simulink model "complete_plant"  (R2022a)
settings: Solver=VariableStepAuto  StartTime=0.0  StopTime=15  RelTol=1e-3
values from neighbouring files (symbols this model uses):
  a = Simulink.Parameter(1.14)    [startup.m]
  A1 = Simulink.Parameter(39.8344)    [startup.m]
  A2 = Simulink.Parameter(813.0780)    [startup.m]
  b = Simulink.Parameter(-0.03291)    [startup.m]
  B1 = Simulink.Parameter(0.000001287)    [startup.m]
  B2 = Simulink.Parameter(-0.002325)    [startup.m]
  B3 = Simulink.Parameter(3.797)    [startup.m]
  c = Simulink.Parameter(-1.14)    [startup.m]
  C1 = Simulink.Parameter(-0.000000002541)    [startup.m]
  C2 = Simulink.Parameter(0.000005279)    [startup.m]
  C3 = Simulink.Parameter(-0.003943)    [startup.m]
  C4 = Simulink.Parameter(3.634)    [startup.m]
  C_param = Simulink.Parameter([0 13757.41 21278.97 26666.02 30253.47 30313.18 30313.18])    [startup.m]
  d = Simulink.Parameter(-1.027)    [startup.m]
  driver_gain = 0.4    [startup.m]
  FZ_C = Simulink.Parameter([0 204.13 427.04 668.1 895.72 1124.40 1324.40])    [startup.m]
  gr = Simulink.Parameter([6.63043, 6.63043, 7.95652, 7.95652])    [startup.m]
  I = 15    [startup.m]
  inch2mm = Simulink.Parameter(25.4)    [startup.m]
  J_z = Simulink.Parameter(75)    [startup.m]
  k_limit = Simulink.Parameter(3.461)    [startup.m]
  Ku = Simulink.Parameter(0.24 / g.Value)    [startup.m]
  l = Simulink.Parameter([0.7922471, 0.7828529])    [startup.m]
  max_yaw_field = Simulink.Parameter([1.34 1.34 1.34 1.66 1.14 1.24 0.754 0.849 0.85 0.85])    [startup.m]
  min_speed_regen = Simulink.Parameter(85)    [startup.m]
  motor_efficiency = Simulink.Parameter([0.85, 0.85, 0.85, 0.85])    [startup.m]
  motor_limit_power = Simulink.Parameter([0, 0, 15000, 15000])    [startup.m]
  motor_limit_torque = Simulink.Parameter([-25, 25])    [startup.m]
  mu_factor = Simulink.Parameter(2/3)    [startup.m]
  P = 1    [startup.m]
  RE = Simulink.Parameter(0.2228169203)    [startup.m]
  s = Simulink.Parameter([0.647895, 0.62102])    [startup.m]
  S1 = Simulink.Parameter(7 * (10^(-5)))    [startup.m]
  S2 = Simulink.Parameter(-0.0038)    [startup.m]
  S3 = Simulink.Parameter(0.6535)    [startup.m]
  S4 = Simulink.Parameter(0.1061)    [startup.m]
  steer_slope = Simulink.Parameter(0.0111)    [startup.m]
  T = 0    [startup.m]
  T2F = Simulink.Parameter(single([29 29 35 35]))    [startup.m]
  tau = Simulink.Parameter(0)    [startup.m]
  time_delay = 0.022    [startup.m]
  V_target = Simulink.Parameter([0 3 6 9 12 15 18 21 25 31])    [startup.m]
undefined symbols (not defined in the file or in its folder): Ag, brake_pressure, DiscIntNeverNeededParam, driver_input, FZ, omega, power_limits, psi, rdot, shock_displacement, shock_velocity, steering_angle, Vg, y, yaw
libraries: fl_lib x20, nesl_utility x12, sdl_lib x4, slpidlib x2, autolibdatasheetbattery x1, autolibmappedmotor x1, vehdynlibtire x1, simulink x1, autolibshared x1, vehdynlibviscommon x1
(part 2 of 3)

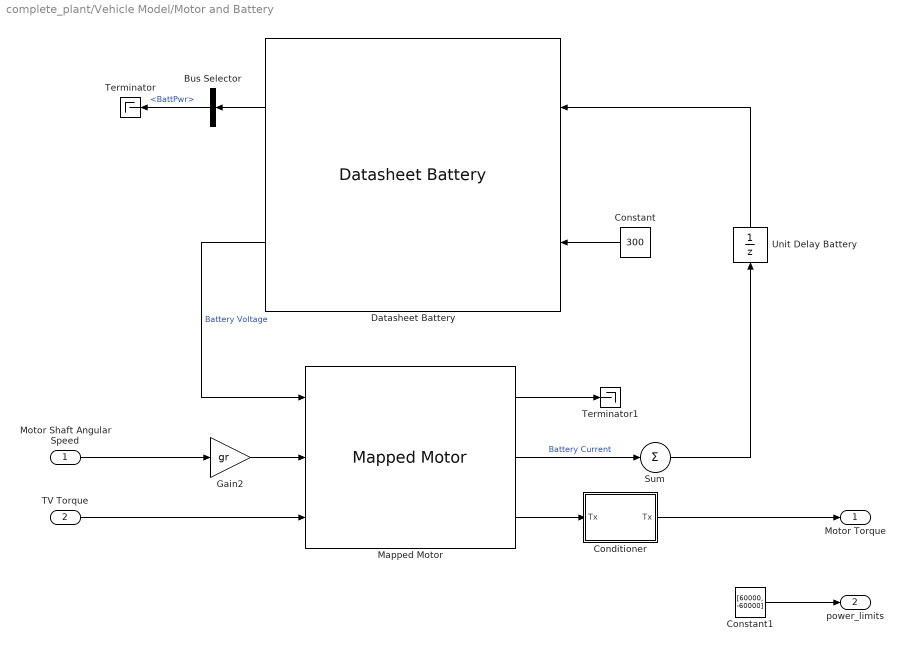
== system complete_plant/Vehicle Model/Motor and Battery ==
  Motor Shaft Angular Speed : Inport
  TV Torque : Inport  Port=2
  Bus Selector : BusSelector  OutputSignals=BattPwr
  Conditioner : MATLAB Function  TreatAsAtomicUnit=on  SystemSampleTime=0.0005
  Constant : Constant  Value=300
  Constant1 : Constant  Value=[60000, -60000]
  Datasheet Battery : autolibdatasheetbattery/Datasheet Battery  CapacityCtrl=Parameter  OutputVlt=Unfiltered  BattChargeMax=16  Em=[2.8 3.228 3.284 3.361 3.408 3.427 3.472 3.477 3.493 3.504 3.516 3.528 3.537 3.545 3.555 3.561 3.566 3.576 3.587 3.589 3.594 3.6 3.608 3.61 3.616 3.619 3.626 3.632 3.637 3.64 3.645 3.646 3.652 3.655 3.658 3.661 3.664 3.668 3.673 3.678 3.68 3.681 3.686 3.692 3.699 3.702 3.705 3.71 3.717 3.723 3.728 3.733 3.735 3.742 3.749 3.755 3.761 3.768 3.773 3.78 3.791 3.798 3.798 3.814 3.818 3.825 3.841 3.846 3.855 3.863 3.877 3.885 3.894 3.907 3.919 3.926 3.935 3.944 3.954 3.964 3.974 3.988 3.998 4.014 4.029 4.034 4.047 4.065 4.074 4.086 4.097 4.131 4.126 4.138 4.15 4.18 4.174 4.187 4.207 4.231 4.221]  CapLUTBp=[0 0.01 0.02 0.03 0.04 0.05 0.06 0.07 0.08 0.09 0.1 0.11 0.12 0.13 0.14 0.15 0.16 0.17 0.18 0.19 0.2 0.21 0.22 0.23 0.24 0.25 0.26 0.27 0.28 0.29 0.3 0.31 0.32 0.33 0.34 0.35 0.36 0.37 0.38 0.39 0.4 0.41 0.42 0.43 0.44 0.45 0.46 0.47 0.48 0.49 0.5 0.51 0.52 0.53 0.54 0.55 0.56 0.57 0.58 0.59 0.6 0.61 0.62 0.63 0.64 0.65 0.66 0.67 0.68 0.69 0.7 0.71 0.72 0.73 0.74 0.75 0.76 0.77 0.78 0.79 0.8 0.81 0.82 0.83 0.84 0.85 0.86 0.87 0.88 0.89 0.9 0.91 0.92 0.93 0.94 0.95 0.96 0.97 0.98 0.99 1]  RInt=[0.008846 0.009319 0.009027 0.00847 0.01032 0.01314;0.006389 0.006554 0.005553 0.005525 0.006043 0.007805;0.004364 0.004101 0.00406 0.003452 0.003846 0.004517;0.002031 0.002563 0.002532 0.00246 0.002716 0.003047;0.001443 0.001825 0.001795 0.001778 0.001924 0.002234;0.0005603 0.0007192 0.0006887 0.0007557 0.0007355 0.001014;0.001028 0.001338 0.001 0.001536 0.001546 0.002789]  BattTempBp=[243.1 253.1 263.1 273.1 283.1 298.1 313.1]  CapSOCBp=[0 0.2 0.4 0.6 0.8 1]  Ns=80  Np=4  BattCapInit=16  Tc=1/1000  Vinit=4.221  RefBlkName='autolibdatasheetbattery/Datasheet Battery'
      settings: SourceProductBaseCode=PW
  Gain2 : Gain  Gain=gr
  Mapped Motor : autolibmappedmotor/Mapped Motor  port_config=Speed  param_by=Tabulated torque-speed envelope  w_t=max_rpm  T_t=max_torque  torque_max=.1  power_max=30  Tc=0.002  param_loss=Tabulated efficiency data  eff=100  w_eff=375  T_eff=0.08  Piron=0  Pbase=0  w_eff_bp=rpm_sweep  T_eff_bp=torque_sweep  Temp_eff_bp=[233.15 293.15 373.15]  losses_table=[1.49 1.67 2.21 3.10; 0.42 0.69 1.14 2.03; 0.06 0.24 0.78 1.68; 0.42 0.69 1.14 2.03; 1.49 1.67 2.21 3.10]  losses_table_3d=cat(3,[1.49 1.67 2.21 3.10; 0.42 0.69 1.14 2.03; 0.06 0.24 0.78 1.68; 0.42 0.69 1.14 2.03; 1.49 1.67 2.21 3.10],[1.49 1.67 2.21 3.10; 0.42 0.69 1.14 2.03; 0.06 0.24 0.78 1.68; 0.42 0.69 1.14 2.03; 1.49 1.67 2.21 3.10],[1.49 1.67 2.21 3.10; 0.42 0.69 1.14 2.03; 0.06 0.24 0.78 1.68; 0.42 0.69 1.14 2.03; 1.49 1.67 2.21 3.10])  efficiency_table=efficiency_grid  efficiency_table_3d=cat(3,[95 95 95 95; 95 95 95 95; 95 95 95 95; 95 95 95 95; 95 95 95 95],[95 95 95 95; 95 95 95 95; 95 95 95 95; 95 95 95 95; 95 95 95 95],[95 95 95 95; 95 95 95 95; 95 95 95 95; 95 95 95 95; 95 95 95 95])  J=5e-6  b=1e-5  omega_o=0  T_t_extended=[0 0.947 1.252 1.562 1.875 2.191 2.511 2.834 3.161 3.491 3.824 4.16 4.499 4.84 5.185 5.532 5.882 6.234 6.589 6.946 7.305 7.666 8.029 8.395 8.762 9.131 9.501 10.247 10.622 10.999 11.376 11.755 12.135 12.516 12.897 13.28 13.663 14.047 14.431 14.815 15.2 15.586 15.971 16.356 16.742 17.127 17.512 17.897 18.281 18.665 19.048 19.431 19.813 20.194 20.574 20.953 21.331 21.708 22.084 22.458 22.83 23.202 23.571 23.939 24.305 24.669 25 25 25 24.669 24.305 23.939 23.571 23.202 22.83 22.458 22.084 21.708 21.331 20.953 20.574 20.194 19.813 19.431 19.048 18.665 18.281 17.897 17.512 17.127 16.742 16.356 15.971 15.586 15.2 14.815 14.431 14.047 13.663 13.28 12.897 12.516 12.135 11.755 11.376 10.999 10.622 10.247 9.501 9.131 8.762 8.395 8.029 7.666 7.305 6.946 6.589 6.234 5.882 5.532 5.185 4.84 4.499 4.16 3.824 3.491 3.161 2.834 2.511 2.191 1.875 1.562 1.252 0.947 0]  w_t_extended=[-1138.429400556 -1112.773060581 -1105.8091968735 -1098.950052921 -1092.2165726745 -1085.5982841585 -1079.095187373 -1072.6968103425 -1066.4136250425 -1060.2351594975 -1054.1614137075 -1048.202859648 -1042.3490253435 -1036.5894388185 -1030.945044024 -1025.394897009 -1019.9389977735 -1014.587818293 -1009.330886592 -1004.1682026705 -999.0997665285 -994.125578166 -989.245637583 -984.449472804 -979.7475558045 -975.129414609 -970.5950492175 -961.7776458465 -957.494607867 -953.2953456915 -949.1693873445 -945.116732826 -941.1478541115 -937.2522792255 -933.4195361925 -929.6705689635 -925.9844335875 -922.37160204 -918.832074321 -915.355378455 -911.941514442 -908.590482282 -905.302281975 -902.076913521 -898.9039049445 -895.793728221 -892.735911375 -889.740926382 -886.7983012665 -883.9080360285 -881.070130668 -878.2741132095 -875.5304556285 -872.839157925 -870.1897481235 -867.582226224 -865.0165922265 -862.492846131 -860.0109879375 -857.571017646 -855.162463281 -852.795796818 -850.4605462815 -848.1567116715 -845.8947649635 -843.6537622065 -841.626809470934 0 841.626809470934 843.6537622065 845.8947649635 848.1567116715 850.4605462815 852.795796818 855.162463281 857.571017646 860.0109879375 862.492846131 865.0165922265 867.582226224 870.1897481235 872.839157925 875.5304556285 878.2741132095 881.070130668 883.9080360285 886.7983012665 889.740926382 892.735911375 895.793728221 898.9039049445 902.076913521 905.302281975 908.590482282 911.941514442 915.355378455 918.832074321 922.37160204 925.9844335875 929.6705689635 933.4195361925 937.2522792255 941.1478541115 945.116732826 949.1693873445 953.2953456915 957.494607867 961.7776458465 970.5950492175 975.129414609 979.7475558045 984.449472804 989.245637583 994.125578166 999.0997665285 1004.1682026705 1009.330886592 1014.587818293 1019.9389977735 1025.394897009 1030.945044024 1036.5894388185 1042.3490253435 1048.202859648 1054.1614137075 1060.2351594975 1066.4136250425 1072.6968103425 1079.095187373 1085.5982841585 1092.2165726745 1098.950052921 1105.8091968735 1112.773060581 1138.429400556]  KLossIron=0  KLossCopper=0  x_w_eff_vec=[-1110.029403 -1099.5574275 -1089.085452 -1078.6134765 -1068.141501 -1057.6695255 -1047.19755 -1036.7255745 -1026.253599 -1015.7816235 -1005.309648 -994.8376725 -984.365697 -973.8937215 -963.421746 -952.9497705 -942.477795 -932.0058195 -921.533844 -911.0618685 -900.589893 -890.1179175 -879.645942 -869.1739665 -858.701991 -848.2300155 -837.75804 -827.2860645 -816.814089 -806.3421135 -795.870138 -785.3981625 -774.926187 -764.4542115 -753.982236 -743.5102605 -733.038285 -722.5663095 -712.094334 -701.6223585 -691.150383 -680.6784075 -670.206432 -659.7344565 -649.262481 -638.7905055 -628.31853 -617.8465545 -607.374579 -596.9026035 -586.430628 -575.9586525 -565.486677 -555.0147015 -544.542726 -534.0707505 -523.598775 -513.1267995 -502.654824 -492.1828485 -481.710873 -471.2388975 -460.766922 -450.2949465 -439.822971 -429.3509955 -418.87902 -408.4070445 -397.935069 -387.4630935 -376.991118 -366.5191425 -356.047167 -345.5751915 -335.103216 -324.6312405 -314.159265 -303.6872895 -293.215314 -282.7433385 -272.271363 -261.7993875 -251.327412 -240.8554365 -230.383461 -219.9114855 -209.43951 -198.9675345 -188.495559 -178.0235835 -167.551608 -157.0796325 -146.607657 -136.1356815 -125.663706 -115.1917305 -104.719755 -94.2477795 -83.775804 -73.3038285 -62.831853 -52.3598775 -41.887902 -31.4159265 -20.943951 -10.4719755 0 10.4719755 20.943951 31.4159265 41.887902 52.3598775 62.831853 73.3038285 83.775804 94.2477795 104.719755 115.1917305 125.663706 136.1356815 146.607657 157.0796325 167.551608 178.0235835 188.495559 198.9675345 209.43951 219.9114855 230.383461 240.8554365 251.327412 261.7993875 272.271363 282.7433385 293.215314 303.6872895 314.159265 324.6312405 335.103216 345.5751915 356.047167 366.5191425 376.991118 387.4630935 397.935069 408.4070445 418.87902 429.3509955 439.822971 450.2949465 460.766922 471.2388975 481.710873 492.1828485 502.654824 513.1267995 523.598775 534.0707505 544.542726 555.0147015 565.486677 575.9586525 586.430628 596.9026035 607.374579 617.8465545 628.31853 638.7905055 649.262481 659.7344565 670.206432 680.6784075 691.150383 701.6223585 712.094334 722.5663095 733.038285 743.5102605 753.982236 764.4542115 774.926187 785.3981625 795.870138 806.3421135 816.814089 827.2860645 837.75804 848.2300155 858.701991 869.1739665 879.645942 890.1179175 900.589893 911.0618685 921.533844 932.0058195 942.477795 952.9497705 963.421746 973.8937215 984.365697 994.8376725 1005.309648 1015.7816235 1026.253599 1036.7255745 1047.19755 1057.6695255 1068.141501 1078.6134765 1089.085452 1099.5574275 1110.029403]  x_T_eff_vec=[-25 -24.9 -24.8 -24.7 -24.6 -24.5 -24.4 -24.3 -24.2 -24.1 -24 -23.9 -23.8 -23.7 -23.6 -23.5 -23.4 -23.3 -23.2 -23.1 -23 -22.9 -22.8 -22.7 -22.6 -22.5 -22.4 -22.3 -22.2 -22.1 -22 -21.9 -21.8 -21.7 -21.6 -21.5 -21.4 -21.3 -21.2 -21.1 -21 -20.9 -20.8 -20.7 -20.6 -20.5 -20.4 -20.3 -20.2 -20.1 -20 -19.9 -19.8 -19.7 -19.6 -19.5 -19.4 -19.3 -19.2 -19.1 -19 -18.9 -18.8 -18.7 -18.6 -18.5 -18.4 -18.3 -18.2 -18.1 -18 -17.9 -17.8 -17.7 -17.6 -17.5 -17.4 -17.3 -17.2 -17.1 -17 -16.9 -16.8 -16.7 -16.6 -16.5 -16.4 -16.3 -16.2 -16.1 -16 -15.9 -15.8 -15.7 -15.6 -15.5 -15.4 -15.3 -15.2 -15.1 -15 -14.9 -14.8 -14.7 -14.6 -14.5 -14.4 -14.3 -14.2 -14.1 -14 -13.9 -13.8 -13.7 -13.6 -13.5 -13.4 -13.3 -13.2 -13.1 -13 -12.9 -12.8 -12.7 -12.6 -12.5 -12.4 -12.3 -12.2 -12.1 -12 -11.9 -11.8 -11.7 -11.6 -11.5 -11.4 -11.3 -11.2 -11.1 -11 -10.9 -10.8 -10.7 -10.6 -10.5 -10.4 -10.3 -10.2 -10.1 -10 -9.9 -9.8 -9.7 -9.6 -9.5 -9.4 -9.3 -9.2 -9.1 -9 -8.9 -8.8 -8.7 -8.6 -8.5 -8.4 -8.3 -8.2 -8.1 -8 -7.9 -7.8 -7.7 -7.6 -7.5 -7.4 -7.3 -7.2 -7.1 -7 -6.9 -6.8 -6.7 -6.6 -6.5 -6.4 -6.3 -6.2 -6.1 -6 -5.9 -5.8 -5.7 -5.6 -5.5 -5.4 -5.3 -5.2 -5.1 -5 -4.9 -4.8 -4.7 -4.6 -4.5 -4.4 -4.3 -4.2 -4.1 -4 -3.9 -3.8 -3.7 -3.6 -3.5 -3.4 -3.3 -3.2 -3.1 -3 -2.9 -2.8 -2.7 -2.6 -2.5 -2.4 -2.3 -2.2 -2.1 -2 -1.9 -1.8 -1.7 -1.6 -1.5 -1.4 -1.3 -1.2 -1.1 -1 -0.9 -0.8 -0.7 -0.6 -0.5 -0.4 -0.3 -0.2 -0.1 0 0.1 0.2 0.3 0.4 0.5 0.6 0.7 0.8 0.9 1 1.1 1.2 1.3 1.4 1.5 1.6 1.7 1.8 1.9 2 2.1 2.2 2.3 2.4 2.5 2.6 2.7 2.8 2.9 3 3.1 3.2 3.3 3.4 3.5 3.6 3.7 3.8 3.9 4 4.1 4.2 4.3 4.4 4.5 4.6 4.7 4.8 4.9 5 5.1 5.2 5.3 5.4 5.5 5.6 5.7 5.8 5.9 6 6.1 6.2 6.3 6.4 6.5 6.6 6.7 6.8 6.9 7 7.1 7.2 7.3 7.4 7.5 7.6 7.7 7.8 7.9 8 8.1 8.2 8.3 8.4 8.5 8.6 8.7 8.8 8.9 9 9.1 9.2 9.3 9.4 9.5 9.6 9.7 9.8 9.9 10 10.1 10.2 10.3 10.4 10.5 10.6 10.7 10.8 10.9 11 11.1 11.2 11.3 11.4 11.5 11.6 11.7 11.8 11.9 12 12.1 12.2 12.3 12.4 12.5 12.6 12.7 12.8 12.9 13 13.1 13.2 13.3 13.4 13.5 13.6 13.7 13.8 13.9 14 14.1 14.2 14.3 14.4 14.5 14.6 14.7 14.8 14.9 15 15.1 15.2 15.3 15.4 15.5 15.6 15.7 15.8 15.9 16 16.1 16.2 16.3 16.4 16.5 16.6 16.7 16.8 16.9 17 17.1 17.2 17.3 17.4 17.5 17.6 17.7 17.8 17.9 18 18.1 18.2 18.3 18.4 18.5 18.6 18.7 18.8 18.9 19 19.1 19.2 19.3 19.4 19.5 19.6 19.7 19.8 19.9 20 20.1 20.2 20.3 20.4 20.5 20.6 20.7 20.8 20.9 21 21.1 21.2 21.3 21.4 21.5 21.6 21.7 21.8 21.9 22 22.1 22.2 22.3 22.4 22.5 22.6 22.7 22.8 22.9 23 23.1 23.2 23.3 23.4 23.5 23.6 23.7 23.8 23.9 24 24.1 24.2 24.3 24.4 24.5 24.6 24.7 24.8 24.9 25]  x_tmp_eff_vec=[-0.09 -0.06 -0.03 0 0.03 0.06 0.09]  x_losses_mat=[2840.43469490031 2805.54744132541 2779.87827049912 2755.63794377818 2733.28147280803 2711.85439946791 2691.24197140587 2671.58877513259 2653.09092346246 2635.0273221516 2618.00782766042 2602.75353700982 2587.04654178768 2572.24579661788 2557.8249286228 2543.77817688114 2530.89179302846 2518.30507115493 2506.11534821342 2494.39397053384 2483.42163017641 2473.65854517521 2463.97979007223 2454.19251617385 2444.74900186613 2434.38941762584 2424.02577848989 2418.02563977851 2412.06569218952 2404.29517518479 2397.44512723314 2390.85220674868 2384.60553603402 2378.95108104658 2373.53020217171 2368.28006687239 2363.00734989155 2358.1662204294 2353.3050369761 2349.21895724092 2345.2633086809 2341.72012007622 2338.58679501067 2335.3809658645 2333.42741875647 2331.43827917154 2329.38942604396 2327.36890336757 2325.26286477187 2323.15588643422 2321.85279256551 2320.45569086905 2318.96446325893 2318.07546934648 2317.46979216667 2316.76053101971 2315.94754163419 2315.93163246198 2316.05712329708 2316.06870267075 2315.96619495001 2316.10738282262 2316.66145037877 2317.09334863559 2317.40287478073 2317.58982555269 2318.21339083604 2319.53316070594 2320.71785979788 2321.76723845613 2322.68104640929 2323.45903276846 2325.03910278562 2327.01714211556 2328.84573681222 2330.52457939056 2332.05336152146 2333.43177402878 2334.6595068864 2336.99421292983 2339.33774137948 2341.51697955451 2343.53155456892 2345.38109240743 2347.06521792118 2348.58355482343 2349.93572568528 2352.56915552233 2355.22622344414 2357.70089624007 2359.99271294185 2362.10121102651 2364.02592640988 2365.76639344001 2367.3221448905 2368.69271195385 2370.28402549494 2373.03179176203 2375.57628226626 2377.91692391904 2380.05314147556 2381.98435752456 2383.70999247813 2385.22946456146 2386.54218980253 2387.64758202168 2388.54505282122 2389.2340115749 2390.39858396493 2392.57021654128 2394.51210477741 2396.22352041458 2397.70373211284 2398.95200543468 2399.96760282866 2400.7497836128 2401.29780395804 2401.61091687151 2401.6883721796 2401.52941651112 2401.13329328017 2400.49924266899 2399.62650161072 2399.31691235657 2400.01959760851 2400.45785502685 2400.63073258304 2400.5372736729 2400.17651708907 2399.5474969933 2398.64924288848 2397.48077959063 2396.04112720045 2394.32930107483 2392.34431179814 2390.08516515324 2387.55086209234 2384.74039870762 2381.6527662016 2378.28695085743 2374.64193400878 2370.71669200961 2366.51019620374 2364.01151523306 2361.45747055781 2358.58844286227 2355.40311978209 2351.90018165219 2348.07830145599 2343.9361447741 2339.47236973265 2334.68562695117 2329.57455948998 2324.13780279725 2318.37398465549 2312.28172512768 2305.85963650287 2299.10632324142 2292.02038191968 2284.60040117421 2276.8449616456 2268.75263592173 2260.32198848061 2251.55157563268 2242.43994546265 2232.98563777082 2223.1871840139 2213.04310724539 2202.55192205531 2192.53352715951 2183.39290654335 2173.8616545439 2163.93786292719 2153.61961101 2142.90496555821 2131.7919806841 2120.2786977426 2108.36314522666 2096.04333866144 2083.31728049752 2070.18296000306 2056.63835315487 2042.68142252842 2028.3101171867 2013.52237256806 1998.31611037286 1982.689238449 1966.63965067636 1950.16522684997 1933.26383256213 1915.93331908323 1898.1715232415 1879.97626730137 1861.34535884079 1842.27659062714 1822.76774049201 1802.81657120464 1782.42083034405 1761.57825016994 1740.28654749222 1718.54342353919 1696.34656382443 1673.69363801224 1650.5822997818 1627.01018668981 1602.9749200318 1578.47410470199 1553.91013607881 1530.09128917938 1505.73387899734 1480.83467203205 1455.39040884597 1429.39780380407 1402.85354481015 1375.75429303985 1348.09668267054 1319.87732060787 1291.09278620896 1261.73963100229 1231.81437840412 1201.3135234314 1170.23353241123 1138.57084268672 1106.32186231915 1073.4829697866 1040.05051367869 1006.02081238763 971.390153795415 936.154794957117 900.310961780193 863.854848699832 826.782618350201 789.090401231568 750.774295373247 711.830365992272 672.254645147765 632.043131390936 ...(+1787558 chars)]  x_losses_mat_3d=[37.8947368421052 25.2631578947368 12.6315789473684 0 12 24 36;18.9473684210526 12.6315789473684 6.3157894736842 0 5.99999999999999 12 18;0 0 0 0 0 0 0;18 12 5.99999999999999 0 6.3157894736842 12.6315789473684 18.9473684210526;36 24 12 0 12.6315789473684 25.2631578947368 37.8947368421052]  CalLossMapData={}  CalLossWithTempMapData={}  aMode=1  RefBlkName='autolibmappedmotor/Mapped Motor'
      settings: SourceProductBaseCode=PW,DR,MT,VE
  Sum : Sum  Inputs=+
  Terminator : Terminator
  Terminator1 : Terminator
  Unit Delay Battery : UnitDelay  SampleTime=0.0005  HasFrameUpgradeWarning=on
  Motor Torque : Outport
  power_limits : Outport  Port=2
  wires:
  Datasheet Battery/1 -> Bus Selector/1
  Constant/1 -> Datasheet Battery/2
  Unit Delay Battery/1 -> Datasheet Battery/1
  Datasheet Battery/2 -> Mapped Motor/1  "Battery Voltage"
  TV Torque/1 -> Mapped Motor/3
  Motor Shaft Angular Speed/1 -> Gain2/1
  Gain2/1 -> Mapped Motor/2
  Mapped Motor/1 -> Terminator1/1
  Mapped Motor/2 -> Sum/1  "Battery Current"
  Sum/1 -> Unit Delay Battery/1
  Bus Selector/1 -> Terminator/1  "<BattPwr>"
  Mapped Motor/3 -> Conditioner/1("Tx ")
  Conditioner/1(Tx) -> Motor Torque/1
  Constant1/1 -> power_limits/1
